simulink subsystem "INS"  (R2025b)
settings: Solver=VariableStepAuto  StartTime=0.0  StopTime=10.0  RelTol=1e-3
libraries: simulink x1
settings Model: Creator=DIEGO  LastModifiedBy=DIEGO

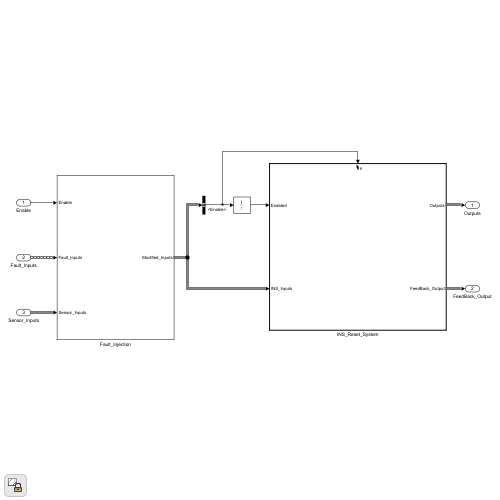
[thumbnail: Simulink's stored preview of the top-level diagram]
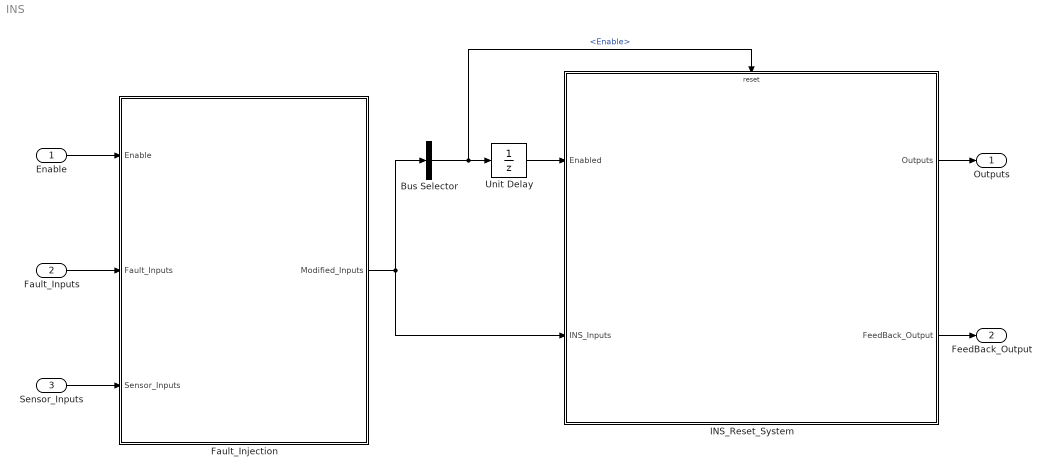
== system INS ==
  Enable : Inport
  Fault_Inputs : Inport  Port=2
  Sensor_Inputs : Inport  Port=3
  Bus Selector : BusSelector  OutputSignals=Enable
  Fault_Injection : Subsystem
  "INS_Reset_System " : Subsystem  TreatAsAtomicUnit=on
  Unit Delay : UnitDelay  SampleTime=-1  HasFrameUpgradeWarning=on
  Outputs : Outport
  FeedBack_Output : Outport  Port=2
  wires:
  Fault_Injection/1(Modified_Inputs) -> "INS_Reset_System "/2(INS_Inputs), Bus Selector/1
  "INS_Reset_System "/2(FeedBack_Output) -> FeedBack_Output/1
  Enable/1 -> Fault_Injection/1(Enable)
  Sensor_Inputs/1 -> Fault_Injection/3(Sensor_Inputs)
  Unit Delay/1 -> "INS_Reset_System "/1(Enabled)
  Bus Selector/1 -> "INS_Reset_System "/Reset, Unit Delay/1  "<Enable>"
  "INS_Reset_System "/1(Outputs) -> Outputs/1
  Fault_Inputs/1 -> Fault_Injection/2(Fault_Inputs)

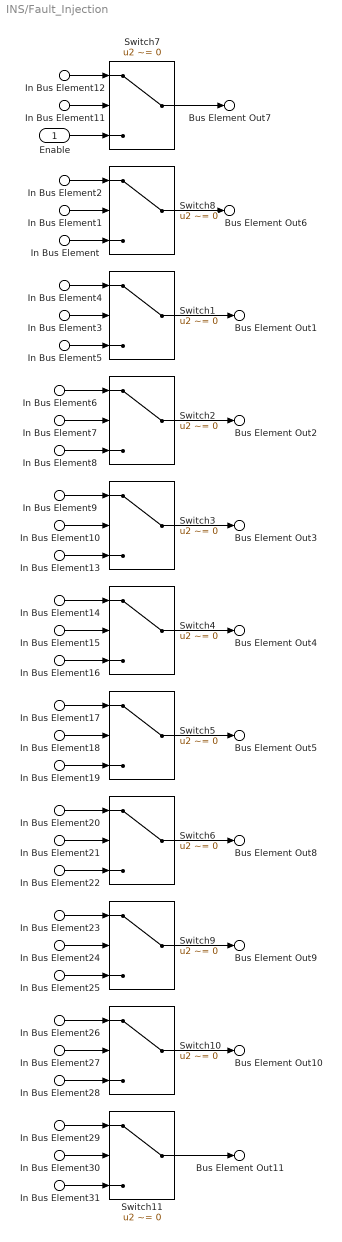
== system INS/Fault_Injection ==
  Enable : Inport
  In Bus Element12 : Inport  Port=2  PortName=Fault_Inputs  Element=Acc_EN
  In Bus Element11 : Inport  Port=2  PortName=Fault_Inputs  Element=Override_Acc_EN
  In Bus Element2 : Inport  Port=2  PortName=Fault_Inputs  Element=Acceleration_X
  In Bus Element3 : Inport  Port=2  PortName=Fault_Inputs  Element=Override_Acceleration_Y
  In Bus Element4 : Inport  Port=2  PortName=Fault_Inputs  Element=Acceleration_Y
  In Bus Element1 : Inport  Port=2  PortName=Fault_Inputs  Element=Override_Acceleration_X
  In Bus Element6 : Inport  Port=2  PortName=Fault_Inputs  Element=Acceleration_Z
  In Bus Element7 : Inport  Port=2  PortName=Fault_Inputs  Element=Override_Acceleration_Z
  In Bus Element9 : Inport  Port=2  PortName=Fault_Inputs  Element=Ground_Speed
  In Bus Element10 : Inport  Port=2  PortName=Fault_Inputs  Element=Override_Ground_Speed
  In Bus Element14 : Inport  Port=2  PortName=Fault_Inputs  Element=Yaw
  In Bus Element15 : Inport  Port=2  PortName=Fault_Inputs  Element=Override_Yaw
  In Bus Element17 : Inport  Port=2  PortName=Fault_Inputs  Element=Pitch
  In Bus Element18 : Inport  Port=2  PortName=Fault_Inputs  Element=Override_Pitch
  In Bus Element20 : Inport  Port=2  PortName=Fault_Inputs  Element=Roll
  In Bus Element21 : Inport  Port=2  PortName=Fault_Inputs  Element=Override_Roll
  In Bus Element23 : Inport  Port=2  PortName=Fault_Inputs  Element=Yaw_Rate
  In Bus Element24 : Inport  Port=2  PortName=Fault_Inputs  Element=Override_Yaw_Rate
  In Bus Element26 : Inport  Port=2  PortName=Fault_Inputs  Element=Pitch_Rate
  In Bus Element27 : Inport  Port=2  PortName=Fault_Inputs  Element=Override_Pitch_Rate
  In Bus Element29 : Inport  Port=2  PortName=Fault_Inputs  Element=Roll_Rate
  In Bus Element30 : Inport  Port=2  PortName=Fault_Inputs  Element=Override_Roll_Rate
  In Bus Element5 : Inport  Port=3  PortName=Sensor_Inputs  Element=Acceleration_Y
  In Bus Element : Inport  Port=3  PortName=Sensor_Inputs  Element=Acceleration_X
  In Bus Element8 : Inport  Port=3  PortName=Sensor_Inputs  Element=Acceleration_Z
  In Bus Element13 : Inport  Port=3  PortName=Sensor_Inputs  Element=Ground_Speed
  In Bus Element16 : Inport  Port=3  PortName=Sensor_Inputs  Element=Yaw
  In Bus Element19 : Inport  Port=3  PortName=Sensor_Inputs  Element=Pitch
  In Bus Element22 : Inport  Port=3  PortName=Sensor_Inputs  Element=Roll
  In Bus Element25 : Inport  Port=3  PortName=Sensor_Inputs  Element=Yaw_Rate
  In Bus Element28 : Inport  Port=3  PortName=Sensor_Inputs  Element=Pitch_Rate
  In Bus Element31 : Inport  Port=3  PortName=Sensor_Inputs  Element=Roll_Rate
  Switch{1..11} (11 alike) : Switch  Criteria=u2 ~= 0  SaturateOnIntegerOverflow=off  InputSameDT=off
  Bus Element Out7 : Outport  PortName=Modified_Inputs  Element=Enable
  Bus Element Out6 : Outport  PortName=Modified_Inputs  Element=Acceleration_X
  Bus Element Out1 : Outport  PortName=Modified_Inputs  Element=Acceleration_Y
  Bus Element Out2 : Outport  PortName=Modified_Inputs  Element=Acceleration_Z
  Bus Element Out3 : Outport  PortName=Modified_Inputs  Element=Ground_Speed
  Bus Element Out4 : Outport  PortName=Modified_Inputs  Element=Yaw
  Bus Element Out5 : Outport  PortName=Modified_Inputs  Element=Pitch
  Bus Element Out8 : Outport  PortName=Modified_Inputs  Element=Roll
  Bus Element Out9 : Outport  PortName=Modified_Inputs  Element=Yaw_Rate
  Bus Element Out10 : Outport  PortName=Modified_Inputs  Element=Pitch_Rate
  Bus Element Out11 : Outport  PortName=Modified_Inputs  Element=Roll_Rate
  wires:
  In Bus Element31/1 -> Switch11/3
  In Bus Element30/1 -> Switch11/2
  In Bus Element29/1 -> Switch11/1
  Switch11/1 -> Bus Element Out11/1
  Switch10/1 -> Bus Element Out10/1
  In Bus Element28/1 -> Switch10/3
  In Bus Element27/1 -> Switch10/2
  In Bus Element26/1 -> Switch10/1
  In Bus Element25/1 -> Switch9/3
  In Bus Element24/1 -> Switch9/2
  In Bus Element23/1 -> Switch9/1
  Switch9/1 -> Bus Element Out9/1
  In Bus Element22/1 -> Switch6/3
  In Bus Element21/1 -> Switch6/2
  In Bus Element20/1 -> Switch6/1
  Switch6/1 -> Bus Element Out8/1
  Switch5/1 -> Bus Element Out5/1
  In Bus Element19/1 -> Switch5/3
  In Bus Element18/1 -> Switch5/2
  In Bus Element17/1 -> Switch5/1
  Switch4/1 -> Bus Element Out4/1
  In Bus Element16/1 -> Switch4/3
  In Bus Element15/1 -> Switch4/2
  In Bus Element14/1 -> Switch4/1
  In Bus Element13/1 -> Switch3/3
  In Bus Element9/1 -> Switch3/1
  In Bus Element10/1 -> Switch3/2
  Switch3/1 -> Bus Element Out3/1
  Switch2/1 -> Bus Element Out2/1
  In Bus Element7/1 -> Switch2/2
  In Bus Element6/1 -> Switch2/1
  In Bus Element8/1 -> Switch2/3
  Enable/1 -> Switch7/3
  In Bus Element11/1 -> Switch7/2
  Switch7/1 -> Bus Element Out7/1
  In Bus Element12/1 -> Switch7/1
  In Bus Element1/1 -> Switch8/2
  In Bus Element/1 -> Switch8/3
  Switch8/1 -> Bus Element Out6/1
  In Bus Element2/1 -> Switch8/1
  In Bus Element5/1 -> Switch1/3
  Switch1/1 -> Bus Element Out1/1
  In Bus Element4/1 -> Switch1/1
  In Bus Element3/1 -> Switch1/2

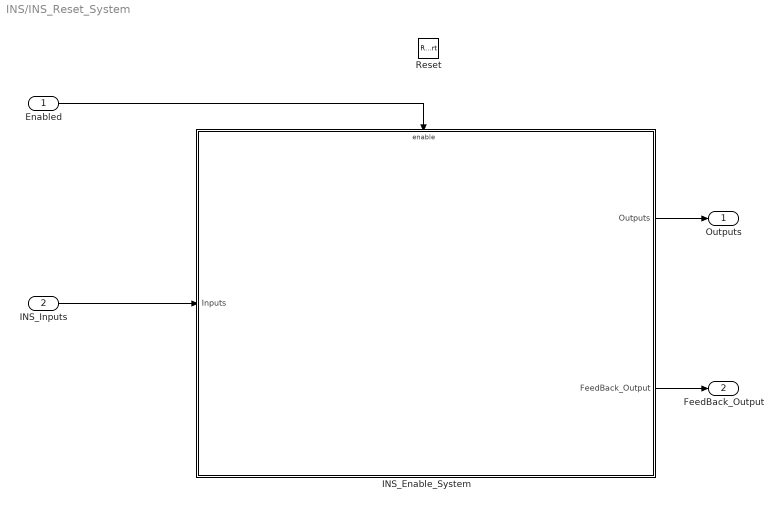
== system INS/INS_Reset_System  ==
  Enabled : Inport
  INS_Inputs : Inport  Port=2
  Reset : ResetPort  DisableCoverage=on  ResetTriggerType=falling
  "INS_Enable_System " : Subsystem  TreatAsAtomicUnit=on
  Outputs : Outport
  FeedBack_Output : Outport  Port=2
  wires:
  Enabled/1 -> "INS_Enable_System "/Enable
  INS_Inputs/1 -> "INS_Enable_System "/1(Inputs)
  "INS_Enable_System "/1(Outputs) -> Outputs/1
  "INS_Enable_System "/2(FeedBack_Output) -> FeedBack_Output/1

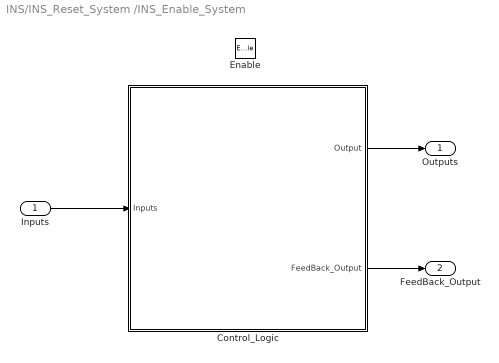
== system INS/INS_Reset_System /INS_Enable_System  ==
  Inputs : Inport
  Enable : EnablePort  StatesWhenEnabling=reset
  Control_Logic : Subsystem
  Outputs : Outport
  FeedBack_Output : Outport  Port=2
  wires:
  Inputs/1 -> Control_Logic/1(Inputs)
  Control_Logic/1(Output) -> Outputs/1
  Control_Logic/2(FeedBack_Output) -> FeedBack_Output/1

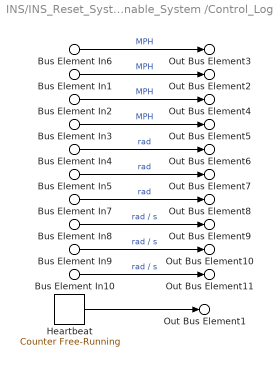
== system INS/INS_Reset_System /INS_Enable_System /Control_Logic ==
  Bus Element In6 : Inport  PortName=Inputs  Element=Acceleration_X
  Bus Element In1 : Inport  PortName=Inputs  Element=Acceleration_Y
  Bus Element In2 : Inport  PortName=Inputs  Element=Acceleration_Z
  Bus Element In3 : Inport  PortName=Inputs  Element=Ground_Speed
  Bus Element In4 : Inport  PortName=Inputs  Element=Yaw
  Bus Element In5 : Inport  PortName=Inputs  Element=Pitch
  Bus Element In7 : Inport  PortName=Inputs  Element=Roll
  Bus Element In8 : Inport  PortName=Inputs  Element=Yaw_Rate
  Bus Element In9 : Inport  PortName=Inputs  Element=Pitch_Rate
  Bus Element In10 : Inport  PortName=Inputs  Element=Roll_Rate
  Heartbeat : simulink/Sources/Counter Free-Running  NumBits=32  tsamp=-1
  Out Bus Element3 : Outport  PortName=Output  Element=Acceleration_X
  Out Bus Element2 : Outport  PortName=Output  Element=Acceleration_Y
  Out Bus Element4 : Outport  PortName=Output  Element=Acceleration_Z
  Out Bus Element5 : Outport  PortName=Output  Element=Ground_Speed
  Out Bus Element6 : Outport  PortName=Output  Element=Yaw
  Out Bus Element7 : Outport  PortName=Output  Element=Pitch
  Out Bus Element8 : Outport  PortName=Output  Element=Roll
  Out Bus Element9 : Outport  PortName=Output  Element=Yaw_Rate
  Out Bus Element10 : Outport  PortName=Output  Element=Pitch_Rate
  Out Bus Element11 : Outport  PortName=Output  Element=Roll_Rate
  Out Bus Element1 : Outport  Port=2  PortName=FeedBack_Output  Element=INS_Heartbeat
  wires:
  Bus Element In10/1 -> Out Bus Element11/1  "rad / s"
  Bus Element In9/1 -> Out Bus Element10/1  "rad / s"
  Bus Element In8/1 -> Out Bus Element9/1  "rad / s"
  Bus Element In7/1 -> Out Bus Element8/1  "rad"
  Bus Element In5/1 -> Out Bus Element7/1  "rad"
  Bus Element In4/1 -> Out Bus Element6/1  "rad"
  Bus Element In3/1 -> Out Bus Element5/1  "MPH"
  Bus Element In2/1 -> Out Bus Element4/1  "MPH"
  Heartbeat/1 -> Out Bus Element1/1
  Bus Element In6/1 -> Out Bus Element3/1  "MPH"
  Bus Element In1/1 -> Out Bus Element2/1  "MPH"
